simulink model "pendel"  (Simulink 7.7)
settings: Solver=ode3  StartTime=0.0  StopTime=10.0  FixedStep=0.01  RelTol=1e-3
values from neighbouring files (symbols this model uses):
  D = 0    [pendel_init.m]
  g = 9.81    [pendel_init.m]
  L = 2    [pendel_init.m]
  m = 1    [pendel_init.m]
  start_dphi = -2    [pendel_init.m]
  start_phi = 90*pi/180    (= 1.57079632679)    [pendel_init.m]
libraries: simulink x2
settings Model: Creator=Alexa  LastModifiedBy=Alexa
settings DebuggingCC: StrictBusMsg=Warning

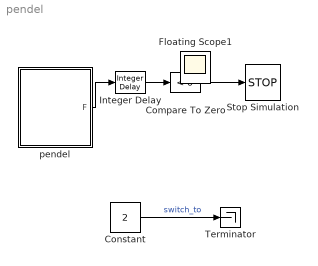
== system pendel ==
  Compare To Zero : simulink/Logic and Bit Operations/Compare To Zero  SystemSampleTime=-1  relop=<  LogicOutDataTypeMode=boolean
  Constant : Constant  Value=2
  Integer Delay : simulink/Discrete/Integer Delay  NumDelays=1  InputProcessing=Inherited  vinit=1  samptime=-1
  Stop Simulation : Stop
  Terminator : Terminator
  pendel : Subsystem
  Floating Scope1 : Scope
      settings: Floating=on  SaveName=ScopeData2
  wires:
  Integer Delay/1 -> Compare To Zero/1
  pendel/1(F) -> Integer Delay/1
  Compare To Zero/1 -> Stop Simulation/1
  Constant/1 -> Terminator/1  "switch_to"

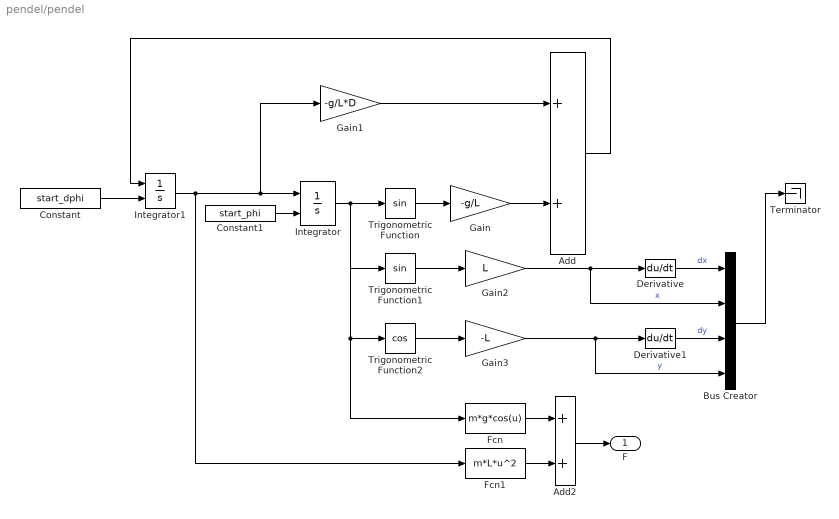
== system pendel/pendel ==
  Add : Sum
  Add2 : Sum
  Bus Creator : BusCreator
  Constant : Constant  Value=start_dphi
  Constant1 : Constant  Value=start_phi
  Derivative : Derivative
  Derivative1 : Derivative
  Fcn : Fcn  Expr=m*g*cos(u)
  Fcn1 : Fcn  Expr=m*L*u^2
  Gain : Gain  Gain=-g/L
  Gain1 : Gain  Gain=-g/L*D
  Gain2 : Gain  Gain=L
  Gain3 : Gain  Gain=-L
  Integrator : Integrator  InitialConditionSource=external  InitialCondition=20
  Integrator1 : Integrator  InitialConditionSource=external
  Terminator : Terminator
  Trigonometric Function : Trigonometry
  Trigonometric Function1 : Trigonometry
  Trigonometric Function2 : Trigonometry  Operator=cos
  F : Outport  OutputWhenDisabled=reset  InitialOutput=[1]
  wires:
  Integrator/1 -> Trigonometric Function1/1, Trigonometric Function2/1, Fcn/1, Trigonometric Function/1
  Trigonometric Function/1 -> Gain/1
  Gain/1 -> Add/2
  Gain1/1 -> Add/1
  Trigonometric Function1/1 -> Gain2/1
  Trigonometric Function2/1 -> Gain3/1
  Gain2/1 -> Bus Creator/2, Derivative/1  "x"
  Integrator1/1 -> Fcn1/1, Gain1/1, Integrator/1
  Constant1/1 -> Integrator/2
  Derivative1/1 -> Bus Creator/3  "dy"
  Fcn/1 -> Add2/1
  Fcn1/1 -> Add2/2
  Add2/1 -> F/1
  Add/1 -> Integrator1/1
  Gain3/1 -> Derivative1/1, Bus Creator/4  "y"
  Derivative/1 -> Bus Creator/1  "dx"
  Constant/1 -> Integrator1/2
  Bus Creator/1 -> Terminator/1
